simulink model "qbot2_post_processing"  (R2020a)
settings: Solver=FixedStepDiscrete  StartTime=0.0  StopTime=P.t(end)  FixedStep=P.dt  RelTol=1e-3  EnableMultiTasking=on
StopFcn:
  | plot_sim(out, P)
settings Model: ExtModeTrigDuration=10000  Creator=divad  LastModifiedBy=divad
settings SolverCC: PositivePriorityOrder=on
settings DataIOCC: SaveOutput=off  SignalLogging=off  DSMLogging=off  SaveTime=off
settings OptimizationCC: LifeSpan=inf
settings DebuggingCC: ArithmeticOperatorsInVariantConditions=warning
settings SFSimCC: SimUseLocalCustomCode=off  CustomCodeUndefinedFunction=UseInterfaceOnly
settings RTWCC: Description=QUARC Win64 Target  SystemTargetFile=quarc_win64.tlc  TemplateMakefile=quarc_default_tmf  RTWUseLocalCustomCode=off
settings CodeAppCC: StateflowObjectComments=on
settings STFCustomTargetCC: TargetPreCompLibLocation=C:\PROGRA~3\QUARC\lib\2020a\win64\release  TargetLangStandard=C99 (ISO)  ConcurrentExecutionCompliant=on  GRTInterface=on  SystemTargetFile=quarc_win64.tlc
settings GRTTargetCC: TargetPreCompLibLocation=C:\PROGRA~3\QUARC\lib\2020a\win64\release  ParMdlRefBuildCompliant=off  CompOptLevelCompliant=off  CombineOutputUpdateFcns=off  MatFileLogging=off  CPPClassGenCompliant=off  GRTInterface=on  UseToolchainInfoCompliant=off  ExtMode=on  ExtModeMexFile=quarc_comm
settings ConfigComp: CovMetricSettings=dswe

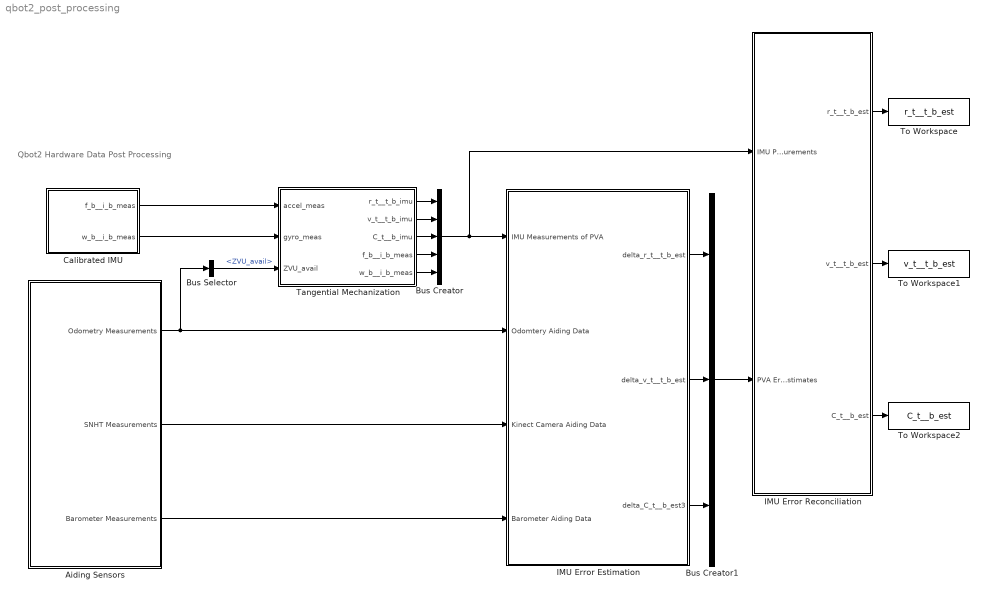
== system qbot2_post_processing ==
  note: Qbot2 Hardware Data Post Processing
  Aiding Sensors : Subsystem
  Bus Creator : BusCreator  Inputs=5
  Bus Creator1 : BusCreator  Inputs=3
  Bus Selector : BusSelector  OutputSignals=ZVU_avail
  Calibrated IMU : Subsystem
  IMU Error Estimation : Subsystem
  IMU Error Reconciliation : Subsystem
  Tangential Mechanization : Subsystem
  To Workspace : ToWorkspace  VariableName=r_t__t_b_est  SampleTime=-1
  To Workspace1 : ToWorkspace  VariableName=v_t__t_b_est  SampleTime=-1
  To Workspace2 : ToWorkspace  VariableName=C_t__b_est  SampleTime=-1
  wires:
  Calibrated IMU/1(f_b__i_b_meas) -> Tangential Mechanization/1(accel_meas)
  Calibrated IMU/2(w_b__i_b_meas) -> Tangential Mechanization/2(gyro_meas)
  Tangential Mechanization/1(r_t__t_b_imu) -> Bus Creator/1
  Tangential Mechanization/2(v_t__t_b_imu) -> Bus Creator/2
  Tangential Mechanization/3(C_t__b_imu) -> Bus Creator/3
  Tangential Mechanization/4(f_b__i_b_meas) -> Bus Creator/4
  Tangential Mechanization/5(w_b__i_b_meas) -> Bus Creator/5
  Bus Creator1/1 -> IMU Error Reconciliation/2(PVA Error Estimates)
  IMU Error Reconciliation/1(r_t__t_b_est) -> To Workspace/1
  IMU Error Reconciliation/2(v_t__t_b_est) -> To Workspace1/1
  IMU Error Reconciliation/3(C_t__b_est) -> To Workspace2/1
  Bus Creator/1 -> IMU Error Estimation/1(IMU Measurements of PVA), IMU Error Reconciliation/1(IMU PVA Measurements)
  Aiding Sensors/1(Odometry Measurements) -> Bus Selector/1, IMU Error Estimation/2(Odomtery Aiding Data)
  Aiding Sensors/2(SNHT Measurements) -> IMU Error Estimation/3(Kinect Camera Aiding Data)
  Aiding Sensors/3(Barometer Measurements) -> IMU Error Estimation/4(Barometer Aiding Data)
  IMU Error Estimation/2(delta_v_t__t_b_est) -> Bus Creator1/2
  IMU Error Estimation/3(delta_C_t__b_est3) -> Bus Creator1/3
  IMU Error Estimation/1(delta_r_t__t_b_est) -> Bus Creator1/1
  Bus Selector/1 -> Tangential Mechanization/3(ZVU_avail)  "<ZVU_avail>"

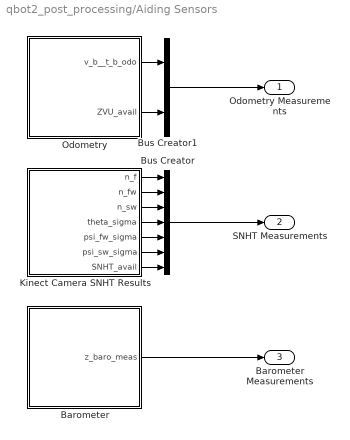
== system qbot2_post_processing/Aiding Sensors ==
  Barometer : Subsystem
  Bus Creator : BusCreator  Inputs=7
  Bus Creator1 : BusCreator  Inputs=2
  Kinect Camera SNHT Results : Subsystem
  Odometry : Subsystem
  Odometry Measurements : Outport
  SNHT Measurements : Outport  Port=2
  Barometer Measurements : Outport  Port=3
  wires:
  Odometry/2(ZVU_avail) -> Bus Creator1/2
  Bus Creator1/1 -> Odometry Measurements/1
  Odometry/1(v_b__t_b_odo) -> Bus Creator1/1
  Barometer/1(z_baro_meas) -> Barometer Measurements/1
  Kinect Camera SNHT Results/1(n_f) -> Bus Creator/1
  Kinect Camera SNHT Results/2(n_fw) -> Bus Creator/2
  Kinect Camera SNHT Results/3(n_sw) -> Bus Creator/3
  Kinect Camera SNHT Results/4(theta_sigma) -> Bus Creator/4
  Kinect Camera SNHT Results/5(psi_fw_sigma) -> Bus Creator/5
  Kinect Camera SNHT Results/6(psi_sw_sigma) -> Bus Creator/6
  Kinect Camera SNHT Results/7(SNHT_avail) -> Bus Creator/7
  Bus Creator/1 -> SNHT Measurements/1

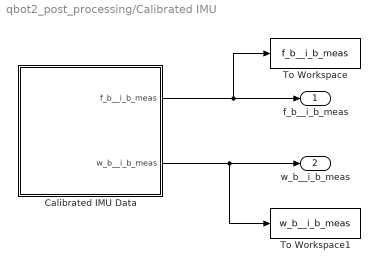
== system qbot2_post_processing/Calibrated IMU ==
  Calibrated IMU Data : MATLAB Function  TreatAsAtomicUnit=on
  To Workspace : ToWorkspace  VariableName=f_b__i_b_meas  SampleTime=-1
  To Workspace1 : ToWorkspace  VariableName=w_b__i_b_meas  SampleTime=-1
  f_b__i_b_meas : Outport
  w_b__i_b_meas : Outport  Port=2
  wires:
  Calibrated IMU Data/2(w_b__i_b_meas) -> To Workspace1/1, w_b__i_b_meas/1
  Calibrated IMU Data/1(f_b__i_b_meas) -> To Workspace/1, f_b__i_b_meas/1

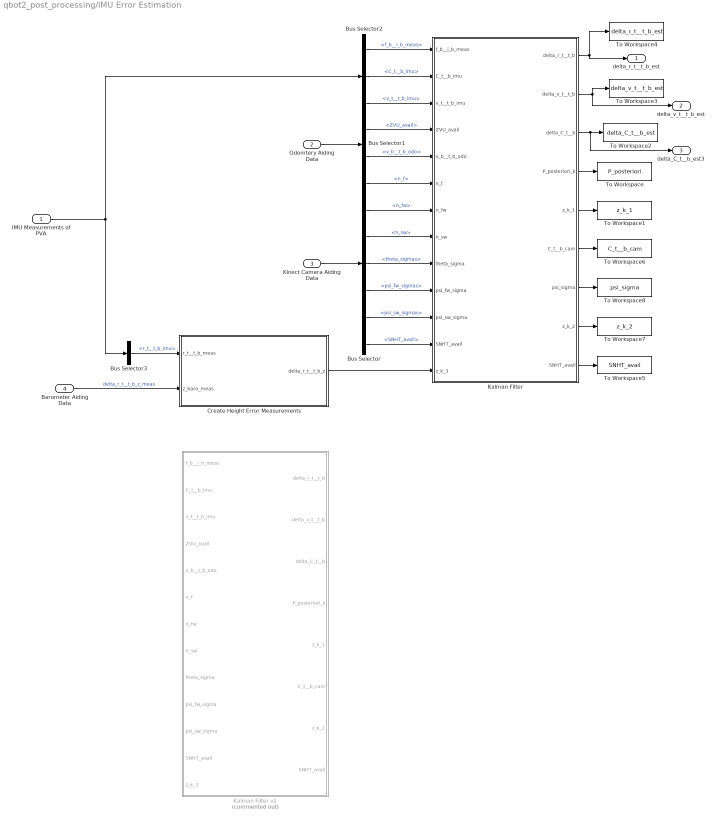
== system qbot2_post_processing/IMU Error Estimation ==
  IMU Measurements of PVA : Inport
  Odomtery Aiding Data : Inport  Port=2
  Kinect Camera Aiding Data : Inport  Port=3
  Barometer Aiding Data : Inport  Port=4
  Bus Selector : BusSelector  OutputSignals=n_f,n_fw,n_sw,theta_sigmas,psi_fw_sigmas,psi_sw_sigmas,SNHT_avail
  Bus Selector1 : BusSelector  OutputSignals=ZVU_avail,v_b__t_b_odo
  Bus Selector2 : BusSelector  OutputSignals=f_b__i_b_meas,C_t__b_imu,v_t__t_b_imu
  Bus Selector3 : BusSelector  OutputSignals=r_t__t_b_imu
  Create Height Error Measurements : Subsystem
  Kalman Filter : MATLAB Function  TreatAsAtomicUnit=on
  Kalman Filter v2 : MATLAB Function  Commented=on  TreatAsAtomicUnit=on
  To Workspace : ToWorkspace  VariableName=P_posteriori  SampleTime=-1
  To Workspace1 : ToWorkspace  VariableName=z_k_1  SampleTime=-1
  To Workspace2 : ToWorkspace  VariableName=delta_C_t__b_est  SampleTime=-1
  To Workspace3 : ToWorkspace  VariableName=delta_v_t__t_b_est  SampleTime=-1
      settings: Save2DSignal=2-D array (concatenate along first dimension)
  To Workspace4 : ToWorkspace  VariableName=delta_r_t__t_b_est  SampleTime=-1
      settings: Save2DSignal=2-D array (concatenate along first dimension)
  To Workspace5 : ToWorkspace  VariableName=SNHT_avail  SampleTime=-1
      settings: Save2DSignal=2-D array (concatenate along first dimension)
  To Workspace6 : ToWorkspace  VariableName=C_t__b_cam  SampleTime=-1
  To Workspace7 : ToWorkspace  VariableName=z_k_2  SampleTime=-1
      settings: Save2DSignal=2-D array (concatenate along first dimension)
  To Workspace8 : ToWorkspace  VariableName=psi_sigma  SampleTime=-1
      settings: Save2DSignal=2-D array (concatenate along first dimension)
  delta_r_t__t_b_est : Outport
  delta_v_t__t_b_est : Outport  Port=2
  delta_C_t__b_est3 : Outport  Port=3
  wires:
  IMU Measurements of PVA/1 -> Bus Selector3/1, Bus Selector2/1
  Barometer Aiding Data/1 -> Create Height Error Measurements/2(z_baro_meas)  "delta_r_t__t_b_z_meas"
  Odomtery Aiding Data/1 -> Bus Selector1/1
  Kinect Camera Aiding Data/1 -> Bus Selector/1
  Bus Selector3/1 -> Create Height Error Measurements/1(r_t__t_b_meas)  "<r_t__t_b_imu>"
  Bus Selector2/1 -> Kalman Filter/1(f_b__i_b_meas)  "<f_b__i_b_meas>"
  Bus Selector2/2 -> Kalman Filter/2(C_t__b_imu)  "<C_t__b_imu>"
  Bus Selector2/3 -> Kalman Filter/3(v_t__t_b_imu)  "<v_t__t_b_imu>"
  Bus Selector1/1 -> Kalman Filter/4(ZVU_avail)  "<ZVU_avail>"
  Bus Selector1/2 -> Kalman Filter/5(v_b__t_b_odo)  "<v_b__t_b_odo>"
  Bus Selector/1 -> Kalman Filter/6(n_f)  "<n_f>"
  Bus Selector/2 -> Kalman Filter/7(n_fw)  "<n_fw>"
  Bus Selector/3 -> Kalman Filter/8(n_sw)  "<n_sw>"
  Bus Selector/4 -> Kalman Filter/9(theta_sigma)  "<theta_sigmas>"
  Bus Selector/5 -> Kalman Filter/10(psi_fw_sigma)  "<psi_fw_sigmas>"
  Bus Selector/6 -> Kalman Filter/11(psi_sw_sigma)  "<psi_sw_sigmas>"
  Bus Selector/7 -> Kalman Filter/12("SNHT_avail ")  "<SNHT_avail>"
  Create Height Error Measurements/1(delta_r_t__t_b_z) -> Kalman Filter/13(z_k_3)
  Kalman Filter/9(SNHT_avail) -> To Workspace5/1
  Kalman Filter/8(z_k_2) -> To Workspace7/1
  Kalman Filter/6(C_t__b_cam) -> To Workspace6/1
  Kalman Filter/5(z_k_1) -> To Workspace1/1
  Kalman Filter/4(P_posteriori_k) -> To Workspace/1
  Kalman Filter/3(delta_C_t__b) -> delta_C_t__b_est3/1, To Workspace2/1
  Kalman Filter/2(delta_v_t__t_b) -> delta_v_t__t_b_est/1, To Workspace3/1
  Kalman Filter/1(delta_r_t__t_b) -> To Workspace4/1, delta_r_t__t_b_est/1
  Kalman Filter/7(psi_sigma) -> To Workspace8/1

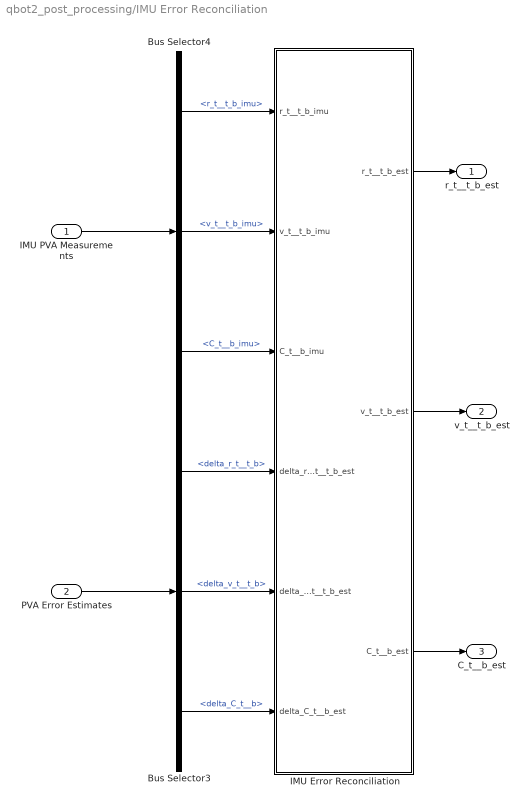
== system qbot2_post_processing/IMU Error Reconciliation ==
  IMU PVA Measurements : Inport
  PVA Error Estimates : Inport  Port=2
  Bus Selector3 : BusSelector  OutputSignals=delta_r_t__t_b,delta_v_t__t_b,delta_C_t__b
  Bus Selector4 : BusSelector  OutputSignals=r_t__t_b_imu,v_t__t_b_imu,C_t__b_imu
  IMU Error Reconciliation : MATLAB Function  TreatAsAtomicUnit=on
  r_t__t_b_est : Outport
  v_t__t_b_est : Outport  Port=2
  C_t__b_est : Outport  Port=3
  wires:
  Bus Selector3/1 -> IMU Error Reconciliation/4(delta_r_t__t_b_est)  "<delta_r_t__t_b>"
  IMU Error Reconciliation/3(C_t__b_est) -> C_t__b_est/1
  Bus Selector4/2 -> IMU Error Reconciliation/2(v_t__t_b_imu)  "<v_t__t_b_imu>"
  Bus Selector4/3 -> IMU Error Reconciliation/3(C_t__b_imu)  "<C_t__b_imu>"
  IMU PVA Measurements/1 -> Bus Selector4/1
  Bus Selector3/2 -> IMU Error Reconciliation/5(delta_v_t__t_b_est)  "<delta_v_t__t_b>"
  IMU Error Reconciliation/2(v_t__t_b_est) -> v_t__t_b_est/1
  Bus Selector4/1 -> IMU Error Reconciliation/1(r_t__t_b_imu)  "<r_t__t_b_imu>"
  Bus Selector3/3 -> IMU Error Reconciliation/6(delta_C_t__b_est)  "<delta_C_t__b>"
  PVA Error Estimates/1 -> Bus Selector3/1
  IMU Error Reconciliation/1(r_t__t_b_est) -> r_t__t_b_est/1

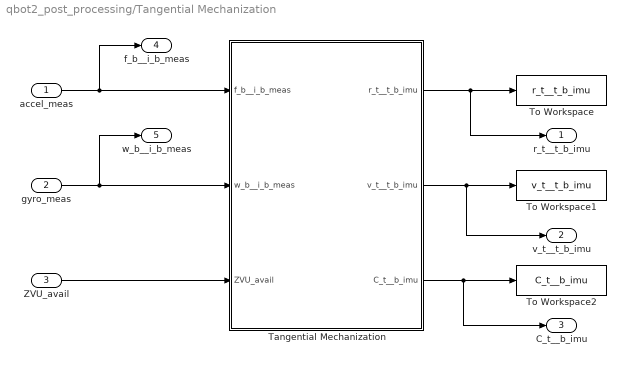
== system qbot2_post_processing/Tangential Mechanization ==
  accel_meas : Inport
  gyro_meas : Inport  Port=2
  ZVU_avail : Inport  Port=3
  Tangential Mechanization : MATLAB Function  TreatAsAtomicUnit=on
  To Workspace : ToWorkspace  VariableName=r_t__t_b_imu  SampleTime=-1
      settings: Save2DSignal=2-D array (concatenate along first dimension)
  To Workspace1 : ToWorkspace  VariableName=v_t__t_b_imu  SampleTime=-1
      settings: Save2DSignal=2-D array (concatenate along first dimension)
  To Workspace2 : ToWorkspace  VariableName=C_t__b_imu  SampleTime=-1
  r_t__t_b_imu : Outport
  v_t__t_b_imu : Outport  Port=2
  C_t__b_imu : Outport  Port=3
  f_b__i_b_meas : Outport  Port=4
  w_b__i_b_meas : Outport  Port=5
  wires:
  Tangential Mechanization/3(C_t__b_imu) -> C_t__b_imu/1, To Workspace2/1
  Tangential Mechanization/2(v_t__t_b_imu) -> v_t__t_b_imu/1, To Workspace1/1
  gyro_meas/1 -> Tangential Mechanization/2(w_b__i_b_meas), w_b__i_b_meas/1
  Tangential Mechanization/1(r_t__t_b_imu) -> r_t__t_b_imu/1, To Workspace/1
  accel_meas/1 -> Tangential Mechanization/1(f_b__i_b_meas), f_b__i_b_meas/1
  ZVU_avail/1 -> Tangential Mechanization/3(ZVU_avail)

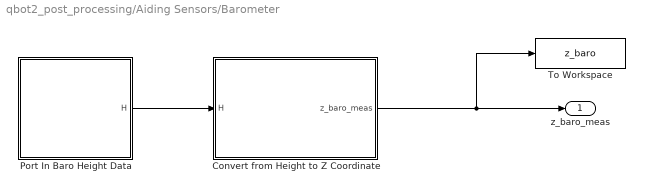
== system qbot2_post_processing/Aiding Sensors/Barometer ==
  Convert from Height to Z Coordinate : MATLAB Function  TreatAsAtomicUnit=on
  Port In Baro Height Data : MATLAB Function  TreatAsAtomicUnit=on
  To Workspace : ToWorkspace  VariableName=z_baro  SampleTime=-1
  z_baro_meas : Outport
  wires:
  Port In Baro Height Data/1(H) -> Convert from Height to Z Coordinate/1(H)
  Convert from Height to Z Coordinate/1(z_baro_meas) -> To Workspace/1, z_baro_meas/1

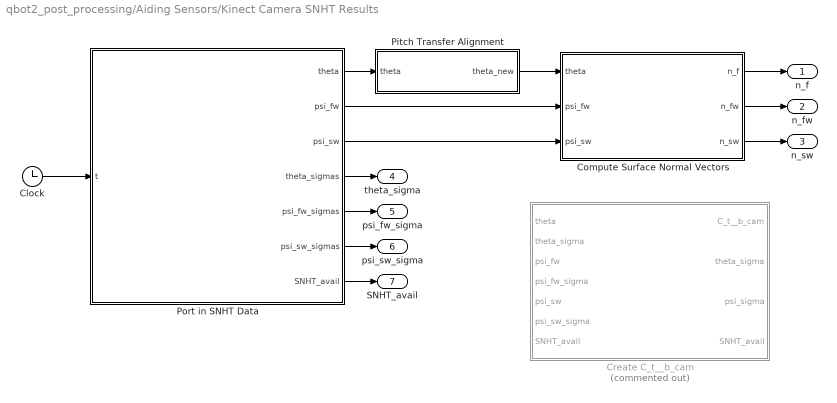
== system qbot2_post_processing/Aiding Sensors/Kinect Camera SNHT Results ==
  Clock : Clock
  Compute Surface Normal Vectors : MATLAB Function  TreatAsAtomicUnit=on
  Create C_t__b_cam : MATLAB Function  Commented=on  TreatAsAtomicUnit=on
  Pitch Transfer Alignment : MATLAB Function  TreatAsAtomicUnit=on
  Port in SNHT Data : MATLAB Function  TreatAsAtomicUnit=on
  n_f : Outport
  n_fw : Outport  Port=2
  n_sw : Outport  Port=3
  theta_sigma : Outport  Port=4
  psi_fw_sigma : Outport  Port=5
  psi_sw_sigma : Outport  Port=6
  SNHT_avail : Outport  Port=7
  wires:
  Port in SNHT Data/1(theta) -> Pitch Transfer Alignment/1(theta)
  Clock/1 -> Port in SNHT Data/1(t)
  Pitch Transfer Alignment/1(theta_new) -> Compute Surface Normal Vectors/1(theta)
  Port in SNHT Data/2(psi_fw) -> Compute Surface Normal Vectors/2(psi_fw)
  Port in SNHT Data/3(psi_sw) -> Compute Surface Normal Vectors/3(psi_sw)
  Port in SNHT Data/7(SNHT_avail) -> SNHT_avail/1
  Port in SNHT Data/6(psi_sw_sigmas) -> psi_sw_sigma/1
  Port in SNHT Data/4(theta_sigmas) -> theta_sigma/1
  Compute Surface Normal Vectors/1(n_f) -> n_f/1
  Compute Surface Normal Vectors/2(n_fw) -> n_fw/1
  Compute Surface Normal Vectors/3(n_sw) -> n_sw/1
  Port in SNHT Data/5(psi_fw_sigmas) -> psi_fw_sigma/1

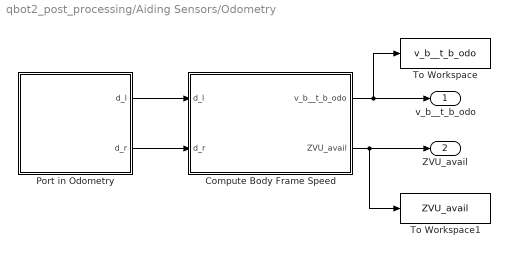
== system qbot2_post_processing/Aiding Sensors/Odometry ==
  Compute Body Frame Speed : MATLAB Function  TreatAsAtomicUnit=on
  Port in Odometry : MATLAB Function  TreatAsAtomicUnit=on
  To Workspace : ToWorkspace  VariableName=v_b__t_b_odo  SampleTime=-1
      settings: Save2DSignal=2-D array (concatenate along first dimension)
  To Workspace1 : ToWorkspace  VariableName=ZVU_avail  SampleTime=-1
  v_b__t_b_odo : Outport
  ZVU_avail : Outport  Port=2
  wires:
  Port in Odometry/2(d_r) -> Compute Body Frame Speed/2(d_r)
  Port in Odometry/1(d_l) -> Compute Body Frame Speed/1(d_l)
  Compute Body Frame Speed/2(ZVU_avail) -> To Workspace1/1, ZVU_avail/1
  Compute Body Frame Speed/1(v_b__t_b_odo) -> To Workspace/1, v_b__t_b_odo/1

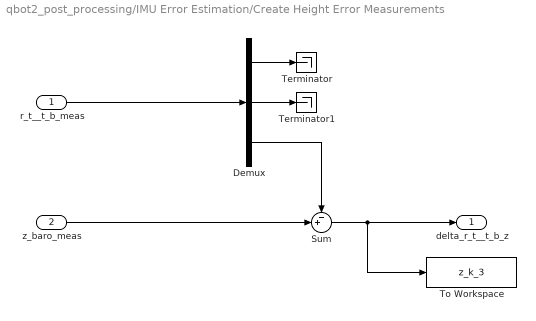
== system qbot2_post_processing/IMU Error Estimation/Create Height Error Measurements ==
  r_t__t_b_meas : Inport
  z_baro_meas : Inport  Port=2
  Demux : Demux  Outputs=3
  Sum : Sum  Inputs=-+|
  Terminator : Terminator
  Terminator1 : Terminator
  To Workspace : ToWorkspace  VariableName=z_k_3  SampleTime=-1
      settings: Save2DSignal=2-D array (concatenate along first dimension)
  delta_r_t__t_b_z : Outport
  wires:
  Demux/3 -> Sum/1
  Demux/2 -> Terminator1/1
  Demux/1 -> Terminator/1
  z_baro_meas/1 -> Sum/2
  Sum/1 -> To Workspace/1, delta_r_t__t_b_z/1
  r_t__t_b_meas/1 -> Demux/1

== matlab function qbot2_post_processing/IMU Error Estimation/Kalman Filter v2 ==
  data: f_b__i_b_meas input; C_t__b_imu input; v_t__t_b_imu input; ZVU_avail input; delta_r_t__t_b output; delta_v_t__t_b output; delta_C_t__b output; v_b__t_b_odo input; n_f input; n_fw input; n_sw input; theta_sigma input; psi_fw_sigma input; psi_sw_sigma input; SNHT_avail input; z_k_3 input; P parameter; P_posteriori_k output; z_k_1 output; C_t__b_cam output; z_k_2 output; SNHT_avail output
function [delta_r_t__t_b, delta_v_t__t_b, delta_C_t__b, P_posteriori_k, ...
          z_k_1, ...
          C_t__b_cam, z_k_2, SNHT_avail] = ...
          IMU_Error_State_Estimation(f_b__i_b_meas, C_t__b_imu, ...
                                     v_t__t_b_imu, ZVU_avail, v_b__t_b_odo, ...
                                     n_f, n_fw, n_sw, theta_sigma, psi_fw_sigma, psi_sw_sigma, SNHT_avail, ...
                                     z_k_3, ...
                                     P)

%% IMU Error State Estimation Function
% Recieves error measurements from the difference between odometry and the
% IMU, and provides estimates of that error.  

persistent x_posteriori_k_1 P_posteriori_k_1 A Q_bar

dt = P.dt;

%**************************************************************************
%% Kalman Filter Prediction Steps
%**************************************************************************

% For first instance only
if (isempty(x_posteriori_k_1))
    
    % Set Initial Values for x and P_______________________________________
    P_0 = diag([5 * pi/180; 5 * pi/180; 5 * pi/180; ... % Initial Attitude Uncertianty (Angle-Axis)
                0.5; 0.5; 0.5; ...                      % Initial Velocity Uncertianty
                0.25; 0.25; 0.25; ...                   % Initial Position Uncertianty 
                10 * P.sigma_n_accel; ...               % Initial Accel Bias Instability Uncertianty
                10 * P.sigma_n_gyro] .^ 2);             % Initial Gyro Bias Instability Uncertianty
            
    x_0 = [dcm2k(P.C_t__b_init); ...                    % First measurement of attitude 
           0; 0; 0;    ...                              % First measurement of velocity error
           0; 0; 0;    ...                              % {t} frame always starts at zero
           P.sigma_n_accel; ...                         % Initialize at the 1-sigma value
           P.sigma_n_gyro];                             % Initialize at the 1-sigma value
       
    x_posteriori_k_1 = x_0;
    P_posteriori_k_1 = P_0;
    
    % Build the Contiuous Time Model_______________________________________
    A = zeros(15, 15);
    
    % Compute A - Fifth Row
    A(13:15, 13:15) = -eye(3) ./ P.cor_time;
    
    % Compute A - Fourth Row
    A(10:12, 10:12) = -eye(3) ./ P.cor_time;
    
    % Compute A - Third Row
    A(7:9, 4:6) = eye(3);
    
    % Compute A - Second Row
    A(4:6, 1:3) = -vec2ss(C_t__b_imu * f_b__i_b_meas);
    A(4:6, 4:6) = -2 .* P.Ohm_t__i_e;
    A(4:6, 10:12) = -C_t__b_imu;

    % Compute the monstrosity A(4:6, 7:9) a.k.a. A_23
    r_e__e_b_hat = P.r_e__e_t; % initial position is always the origin
    [L_b_hat, ~, ~] = xyz2llh(r_e__e_b_hat, P);
    g_0 = Somigliana(L_b_hat, P);
    r_e__e_S = Geo_Radius(L_b_hat, P);
    A(4:6, 7:9) = P.C_e__t' * ((2 * g_0 * r_e__e_b_hat) / ...
                 (r_e__e_S * norm(r_e__e_b_hat)^2)) * ...
                  r_e__e_b_hat' * P.C_e__t;
    
    % Compute A - First Row
    A(1:3, 1:3) = -P.Ohm_t__i_e;
    A(1:3, 13:15) = -C_t__b_imu;
    
    % Define Q_bar_________________________________________________________
    Q_vec = [P.gyro_ARW.^2;   ...        % Attitude Process Noise rad/s
             P.accel_VRW.^2;  ...        % Velocity Process Noise m/s
             zeros(3,1);         ...     % Position Process Noise
             P.sigma_n_accel.^2; ...     % Accel Bias Instability Process Noise m/s
             P.sigma_n_gyro.^2];         % Gyro  Bias Instability Process Noise rad/s
     
    % Allow for a margin of error for tuning     
    Q_fudge_factor = 1;
    
    % Set Q
    Q_bar = diag(Q_fudge_factor .* Q_vec');
    
    % Discritize the Continuous Time Model_________________________________
    F = eye(15) + A*dt;
    Q = (1/2) * ((F*Q_bar*F') + Q_bar) * dt;
    
    % Compute first prediction_____________________________________________
    x_priori_k = F * x_0;
    P_priori_k = (F * P_0 * F') + Q;
    
%__________________________________________________________________________
% All other instances: State Prediction  
else
    
    % Re-compute the time varying arguements of A__________________________

    % Compute A - Second Row
    A(4:6, 1:3) = -vec2ss(C_t__b_imu * f_b__i_b_meas);
    A(4:6, 10:12) = -C_t__b_imu;
    
    % Compute A - First Row
    A(1:3, 13:15) = -C_t__b_imu;
    
    % Discritize the Continuous Time Model_________________________________
    F = eye(15) + A*dt;
    Q = (1/2) * ((F*Q_bar*F') + Q_bar) * dt;
    
    % Compute prediction step
    x_priori_k = (F * x_posteriori_k_1);
    P_priori_k = (F * P_posteriori_k_1 * F') + Q;
    
    % Symmetrisize P
    P_priori_k = (P_priori_k + P_priori_k') / 2;
    
end

%**************************************************************************
%% Compute Kalman Filter Measurements
%**************************************************************************

%__________________________________________________________________________
% Odometry Velocity Error Mesaurement Computation

if (P.aiding_sensor_config == 4) | ...
   (P.aiding_sensor_config == 6) | ...
   (P.aiding_sensor_config == 7)
    
    %- - - - - - - - - - - - - - - - - - - - - - - - - - - - - - - - - - -
    % If a Zero Velocity Update (ZVU) is available
    if (ZVU_avail == 1)
        
        % Then error is simply the measurement
        z_k_1 = -v_t__t_b_imu;
        
        % Uncertianty of Velocity Error is 5 millameters
        R_odo_vec = [0.001, 0.001, 0.001] .^ 2;     
    
    %- - - - - - - - - - - - - - - - - - - - - - - - - - - - - - - - - - - 
    % If a Zero Velocity is NOT Available
    else
        
        % Rotate v_b__t_b_odo with best estimate of attitude
        delta_C_t__b_est = k2dcm(x_priori_k(1:3,1));
        C_t__b_est = C_t__b_imu * delta_C_t__b_est';
        v_t__t_b_odo = C_t__b_est * v_b__t_b_odo;
        delta_v_t__t_b_meas = v_t__t_b_odo - v_t__t_b_imu;
        z_k_1 = delta_v_t__t_b_meas;
        
        % Define R Vector
        R_b_vec = [0.05, 0.01, 0.01] .^ 2;   % Will come back to this!
        
        % Build the R Matrix
        R_odo = C_t__b_imu * diag(R_b_vec) * C_t__b_imu';
        R_odo_vec = [R_odo(1,1), R_odo(2,2), R_odo(3,3)];
        
    end

else
    
    z_k_1 = zeros(3,1);
 
end

%__________________________________________________________________________
% Kinect Camera Attitude Error Measurement Computation

if ((P.aiding_sensor_config == 5) | ...
    (P.aiding_sensor_config == 6) | ...
    (P.aiding_sensor_config == 7))
    
    if (SNHT_avail == 1)
        
        % Compute C_t__b_est
        delta_C_t__b_est = k2dcm(x_priori_k(1:3,1));
        C_t__b_est = C_t__b_imu * delta_C_t__b_est';
        
        % Compute C_t__b_cam
        [C_t__b_cam, psi_sigma, SNHT_avail] = get_C_t__b_cam(n_f, n_fw, n_sw, ...
            psi_fw_sigma, psi_sw_sigma, C_t__b_imu, C_t__b_est);
        
        if (SNHT_avail == 1)
            
            % Define R_e with known sigmas
            R_e = diag([1 * pi/180, theta_sigma, psi_sigma]) .^ 2;
            
            % Create Error in Attitude Measurement
            z_k_2 = dcm2k(C_t__b_cam * C_t__b_imu');
            
            % Compute Jacobian
            [~, pitch, roll] = dcm2ypr(C_t__b_est);
            J = [1, 0, -sin(pitch); ...
                0, cos(roll), sin(roll)*cos(pitch); ...
                0, -sin(roll), cos(roll)*cos(pitch)];
            
            % Convert R_e to R_k
            R_k = J * R_e * J';
            R_k_vec = [R_k(1), R_k(2), R_k(3)];
            
        else
            
            z_k_2 = zeros(3,1);
            R_k_vec = zeros(1,3);
            C_t__b_cam = eye(3);
            
        end
        
        
    else
        
        z_k_2 = zeros(3,1);
        R_k_vec = zeros(1,3);
        C_t__b_cam = eye(3);
        
    end
    
else
    
    z_k_2 = zeros(3,1);
    R_k_vec = zeros(1,3);
    C_t__b_cam = eye(3);
    
end

%**************************************************************************
%% Kalman Filter Measurement Update Steps
%**************************************************************************
% This section is segmented according to the aiding sensor configuration

%__________________________________________________________________________
% If no aiding sensors are included
if (P.aiding_sensor_config == 0)
    
    x_posteriori_k = x_priori_k;
    P_posteriori_k = P_priori_k;

%__________________________________________________________________________
% If any aiding sensor is selected
else
    
    % Create Starting Point
    H = zeros(9,15);
    R_vec = 10^6 * ones(1,9);
    z = zeros(9,1);
    
    % Build H & R & z for Odometry
    if (P.aiding_sensor_config ~= 5)
        if (norm(x_priori_k) <= (10 * pi/180))
            H(4:6,:) = [vec2ss(v_t__t_b_imu), eye(3), zeros(3,9)];
        else
            H(4:6,:) = [zeros(3,3), eye(3), zeros(3,9)];
        end
        R_vec(4:6) = R_odo_vec;
        z(4:6) = z_k_1;
    end
    
    % Build H & R & z for Kinect Camera if present
    if (SNHT_avail == 1)
        H(1:3,:) = [eye(3), zeros(3,12)];
        R_vec(1:3) = R_k_vec;
        z(1:3) = z_k_2;
    end
    
    
    % Build H & R & z for Barometer is present
    if (P.aiding_sensor_config == 7)
        H(9,9) = 1;
        R_vec(9) = 0.3^2;
        z(9) = z_k_3;
    end
    
    
    % Build full R
    R = diag(R_vec);
    
    % Complete full measurement update
    % Kalman Gain Computation
    K = (P_priori_k * H') / (H * P_priori_k * H' + R);
    
    % A Posteriori State and Covariance Update
    x_posteriori_k = x_priori_k + K*(z - H*x_priori_k);
    P_posteriori_k = (eye(15) - K*H) * P_priori_k;
    
    %Symmetrisize P
    P_posteriori_k = (P_posteriori_k + P_posteriori_k') / 2;
    
end

%__________________________________________________________________________
%% Pick-off State Estimates for Function Output

% State Estimates (AVP -> PVA)
delta_x_t__t_b_est = [x_posteriori_k(7:9); ...
                      x_posteriori_k(4:6); ...
                      x_posteriori_k(1:3)];

% Pull Off Position, Velocity, and Attitude Error Separately
delta_r_t__t_b = delta_x_t__t_b_est(1:3);
delta_v_t__t_b = delta_x_t__t_b_est(4:6);
delta_k_t__t_b = delta_x_t__t_b_est(7:9);

% Create and Normalize delta_C_t__b
delta_C_t__b = k2dcm(delta_k_t__t_b);
delta_C_t__b = q2dcm(dcm2q(delta_C_t__b));

%__________________________________________________________________________
%% Save State Estimates for Next Loop

x_posteriori_k_1 = x_posteriori_k;
P_posteriori_k_1 = P_posteriori_k;

end

== matlab function qbot2_post_processing/Aiding Sensors/Kinect Camera SNHT Results/Port in SNHT Data ==
  data: t input; theta output; psi_fw output; psi_sw output; theta_sigmas output; psi_fw_sigmas output; psi_sw_sigmas output; P parameter; SNHT_avail output
function [theta, psi_fw, psi_sw, theta_sigmas, psi_fw_sigmas, psi_sw_sigmas, SNHT_avail] = port_in_SNHT(t, P)

%% Initialize
 persistent k
 
 if (isempty(k))
     k = 1;
 end
 
 %% Port in SNHT Results at 1 Hz
 
 if (mod(t, 1) == 0)
     
     % Pitch Results
     theta = P.theta_meas(k);
     theta_sigmas = P.theta_sigmas(k);
     
     % Front Wall Results
     psi_fw = P.psi_fw_meas(k);
     psi_fw_sigmas = P.psi_fw_sigmas(k);
     
     % Side Wall Results
     psi_sw = P.psi_sw_meas(k);
     psi_sw_sigmas = P.psi_sw_sigmas(k);
     
     % Make SNHT_avail true
     SNHT_avail = 1;
     
     % Increment
     k = k + 1;
     
 else
     
     % Pitch Results
     theta = P.pitch_trans_align;
     theta_sigmas = 45 * pi/180;
     
     % Front Wall Results
     psi_fw = 0;
     psi_fw_sigmas = 45 * pi/180;
     
     % Side Wall Results
     psi_sw = 90;
     psi_sw_sigmas = 45 * pi/180;
     
     % Make SNHT_avail true
     SNHT_avail = 0;
     
 end

 if (t == 0)
     SNHT_avail = 0;
 end

== matlab function qbot2_post_processing/Aiding Sensors/Kinect Camera SNHT Results/Create C_t__b_cam ==
  data: theta input; theta_sigma input; C_t__b_cam output; psi_fw input; psi_fw_sigma input; psi_sw input; psi_sw_sigma input; theta_sigma output; psi_sigma output; SNHT_avail input; SNHT_avail output
function [C_t__b_cam, theta_sigma, psi_sigma, SNHT_avail]  = ...
    create_C_t__b_cam(theta, theta_sigma, psi_fw, psi_fw_sigma, psi_sw, psi_sw_sigma, SNHT_avail)

%% Initialize Caresian Frame Axes
persistent x_b y_b z_b

if (isempty(x_b))
    
    % Define Body Frame Axes
    x_b = [1; 0; 0];
    y_b = [0; 1; 0];
    z_b = [0; 0; 1];
    
end

%% Only Complete when SNHT Results are available
if (SNHT_avail == 1)
    
    % Define normal vectors
    n_f  = [sin(theta); 0; cos(theta)];
    n_fw = [cos(psi_fw); sin(psi_fw); 0];
    n_sw = [-cos(psi_sw); sin(psi_sw); 0];
    
    % Normalize the Normal Vectors
    n_f = n_f / norm(n_f);
    n_fw = n_fw / norm(n_fw);
    n_sw = n_sw / norm(n_sw);
    
    % Define Body Frame Axes from Measurements, and Return Sigmas
    if (psi_fw_sigma <= psi_sw_sigma)
        x_t = n_fw;
        y_t = -(cross(n_fw, n_f));
        z_t = n_f;
        psi_sigma = psi_fw_sigma;
    else
        x_t = cross(n_sw, n_f);
        y_t = n_sw;
        z_t = n_f;
        psi_sigma = psi_sw_sigma;
    end
    
    %% Create C_t__b_cam
    
    % Build DCM
    C_b__t_cam = [dot(x_t, x_b), dot(y_t, x_b), dot(z_t, x_b); ...
                  dot(x_t, y_b), dot(y_t, y_b), dot(z_t, y_b); ...
                  dot(x_t, z_b), dot(y_t, z_b), dot(z_t, z_b)];
    
    C_t__b_cam = C_b__t_cam';
              
    % Normalize
    C_t__b_cam = q2dcm(dcm2q(C_t__b_cam));        

%% When SNHT Result is not Available
else
    
    % Set to default values
    C_t__b_cam = eye(3);
    theta_sigma = 45;
    psi_sigma = 45;
    
end

end

== matlab function qbot2_post_processing/Aiding Sensors/Barometer/Port In Baro Height Data ==
  data: H output; P parameter
function H = port_in_baro_data(P)

%% Initialize
persistent k T_s k_T p_s R g_0

if (isempty(k))
    
    % Initialize k
    k = 1;
    
    % Initialize Pressure to Height Conversion
    T_s = 288.15;
    k_T = 0.0065;
    p_s = 101.325;
    R = 287.058;
    g_0 = 9.0665;

end

%% Convert Pressure to Height
H = (T_s / k_T) * ((P.baro(k)/p_s)^(-R*k_T/g_0) - 1);

% Increment
k = k + 1;

end

== matlab function qbot2_post_processing/Aiding Sensors/Barometer/Convert from Height to Z Coordinate ==
  data: H input; z_baro_meas output; P parameter
function z_baro_meas = convert_H_to_z(H, P)

z_baro_meas = H - P.H_avg;

== matlab function qbot2_post_processing/Aiding Sensors/Kinect Camera SNHT Results/Pitch Transfer Alignment ==
  data: theta input; theta_new output; P parameter
function theta_new  = pitch_transfer_alignment(theta, P)

theta_new = theta - P.pitch_trans_align;

== matlab function qbot2_post_processing/IMU Error Reconciliation/IMU Error Reconciliation ==
  data: r_t__t_b_imu input; r_t__t_b_est output; v_t__t_b_imu input; C_t__b_imu input; v_t__t_b_est output; C_t__b_est output; delta_r_t__t_b_est input; delta_v_t__t_b_est input; delta_C_t__b_est input; P parameter
function [r_t__t_b_est, v_t__t_b_est, C_t__b_est] = ...
    imu_error_reconcile(r_t__t_b_imu, v_t__t_b_imu, C_t__b_imu, ...
                        delta_r_t__t_b_est, delta_v_t__t_b_est, delta_C_t__b_est, P)
       
% No reconciliation for pure imu only
if (P.aiding_sensor_config == 0)
    
    r_t__t_b_est = r_t__t_b_imu;
    v_t__t_b_est = v_t__t_b_imu;
    C_t__b_est = C_t__b_imu;

% Adjust for every other aiding sensor config
else
                    
    % Reconclie Position
    r_t__t_b_est = r_t__t_b_imu + delta_r_t__t_b_est;
    
    % Reconcile Velocity
    v_t__t_b_est = v_t__t_b_imu + delta_v_t__t_b_est;
    
    % Reconclie Attitude
    C_t__b_est = C_t__b_imu * delta_C_t__b_est;

end

== matlab function qbot2_post_processing/Aiding Sensors/Kinect Camera SNHT Results/Compute Surface Normal Vectors ==
  data: theta input; n_f output; psi_fw input; psi_sw input; n_fw output; n_sw output
function [n_f, n_fw, n_sw] = compute_surface_normal_vectors(theta, psi_fw, psi_sw)

% Build Normal Vectors
n_f = [sin(theta); 0; cos(theta)];
n_fw = [cos(psi_fw); sin(psi_fw); 0];
n_sw = [-cos(psi_sw); sin(psi_sw); 0];

end

== matlab function qbot2_post_processing/Calibrated IMU/Calibrated IMU Data ==
  data: f_b__i_b_meas output; w_b__i_b_meas output; P parameter
function [f_b__i_b_meas, w_b__i_b_meas] = IMU_meas(P)

persistent k

if (isempty(k))
    k = 1;
end

% Load Accel Frame
f_b__i_b_meas = P.f_b__i_b_meas(:,k);

% Load Gyro Frame
w_b__i_b_meas = P.w_b__i_b_meas(:,k);

% Index to Next Frame
k = k + 1;

== matlab function qbot2_post_processing/IMU Error Estimation/Kalman Filter ==
  data: f_b__i_b_meas input; C_t__b_imu input; v_t__t_b_imu input; ZVU_avail input; delta_r_t__t_b output; delta_v_t__t_b output; delta_C_t__b output; v_b__t_b_odo input; n_f input; n_fw input; n_sw input; theta_sigma input; psi_fw_sigma input; psi_sw_sigma input; SNHT_avail input; z_k_3 input; P parameter; P_posteriori_k output; z_k_1 output; C_t__b_cam output; psi_sigma output; z_k_2 output; SNHT_avail output
function [delta_r_t__t_b, delta_v_t__t_b, delta_C_t__b, P_posteriori_k, ...
          z_k_1, ...
          C_t__b_cam, psi_sigma, z_k_2, SNHT_avail] = ...
          IMU_Error_State_Estimation(f_b__i_b_meas, C_t__b_imu, ...
                                     v_t__t_b_imu, ZVU_avail, v_b__t_b_odo, ...
                                     n_f, n_fw, n_sw, theta_sigma, psi_fw_sigma, psi_sw_sigma, SNHT_avail, ...
                                     z_k_3, ...
                                     P)

%% IMU Error State Estimation Function
% Recieves error measurements from the difference between odometry and the
% IMU, and provides estimates of that error.  

persistent x_posteriori_k_1 P_posteriori_k_1 A Q_bar

dt = P.dt;

% Normalize C_t__b_est
C_t__b_imu = q2dcm(dcm2q(C_t__b_imu));

%**************************************************************************
%% Kalman Filter Prediction Steps
%**************************************************************************

% For first instance only
if (isempty(x_posteriori_k_1))
    
    % Set Initial Values for x and P_______________________________________
    P_0 = diag([5 * pi/180; 5 * pi/180; 5 * pi/180; ... % Initial Attitude Uncertianty (Angle-Axis)
                0.5; 0.5; 0.5; ...                      % Initial Velocity Uncertianty
                0.25; 0.25; 0.25; ...                   % Initial Position Uncertianty 
                10 * P.sigma_n_accel; ...               % Initial Accel Bias Instability Uncertianty
                10 * P.sigma_n_gyro] .^ 2);             % Initial Gyro Bias Instability Uncertianty
            
    x_0 = [dcm2k(P.C_t__b_init); ...                    % First measurement of attitude 
           0; 0; 0;    ...                              % First measurement of velocity error
           0; 0; 0;    ...                              % {t} frame always starts at zero
           P.sigma_n_accel; ...                         % Initialize at the 1-sigma value
           P.sigma_n_gyro];                             % Initialize at the 1-sigma value
       
    x_posteriori_k_1 = x_0;
    P_posteriori_k_1 = P_0;
    d_prev = 0;
    
    % Build the Contiuous Time Model_______________________________________
    A = zeros(15, 15);
    
    % Compute A - Fifth Row
    A(13:15, 13:15) = -eye(3) ./ P.cor_time;
    
    % Compute A - Fourth Row
    A(10:12, 10:12) = -eye(3) ./ P.cor_time;
    
    % Compute A - Third Row
    A(7:9, 4:6) = eye(3);
    
    % Compute A - Second Row
    A(4:6, 1:3) = -vec2ss(C_t__b_imu * f_b__i_b_meas);
    A(4:6, 4:6) = -2 .* P.Ohm_t__i_e;
    A(4:6, 10:12) = -C_t__b_imu;

    % Compute the monstrosity A(4:6, 7:9) a.k.a. A_23
    r_e__e_b_hat = P.r_e__e_t; % initial position is always the origin
    [L_b_hat, ~, ~] = xyz2llh(r_e__e_b_hat, P);
    g_0 = Somigliana(L_b_hat, P);
    r_e__e_S = Geo_Radius(L_b_hat, P);
    A(4:6, 7:9) = P.C_e__t' * ((2 * g_0 * r_e__e_b_hat) / ...
                 (r_e__e_S * norm(r_e__e_b_hat)^2)) * ...
                  r_e__e_b_hat' * P.C_e__t;
    
    % Compute A - First Row
    A(1:3, 1:3) = -P.Ohm_t__i_e;
    A(1:3, 13:15) = -C_t__b_imu;
    
    % Define Q_bar_________________________________________________________
    Q_vec = [P.gyro_ARW.^2;   ...        % Attitude Process Noise rad/s
             P.accel_VRW.^2;  ...        % Velocity Process Noise m/s
             zeros(3,1);         ...     % Position Process Noise
             P.sigma_n_accel.^2; ...     % Accel Bias Instability Process Noise m/s
             P.sigma_n_gyro.^2];         % Gyro  Bias Instability Process Noise rad/s
     
    % Allow for a margin of error for tuning     
    Q_fudge_factor = 1;
    
    % Set Q
    Q_bar = diag(Q_fudge_factor .* Q_vec');
    
    % Discritize the Continuous Time Model_________________________________
    F = eye(15) + A*dt;
    Q = (1/2) * ((F*Q_bar*F') + Q_bar) * dt;
    
    % Compute first prediction_____________________________________________
    x_priori_k = F * x_0;
    P_priori_k = (F * P_0 * F') + Q;
    
%__________________________________________________________________________
% All other instances: State Prediction  
else
    
    % Re-compute the time varying arguements of A__________________________

    % Compute A - Second Row
    A(4:6, 1:3) = -vec2ss(C_t__b_imu * f_b__i_b_meas);
    A(4:6, 10:12) = -C_t__b_imu;
    
    % Compute A - First Row
    A(1:3, 13:15) = -C_t__b_imu;
    
    % Discritize the Continuous Time Model_________________________________
    F = eye(15) + A*dt;
    Q = (1/2) * ((F*Q_bar*F') + Q_bar) * dt;
    
    % Compute prediction step
    x_priori_k = (F * x_posteriori_k_1);
    P_priori_k = (F * P_posteriori_k_1 * F') + Q;
    
    % Symmetrisize P
    P_priori_k = (P_priori_k + P_priori_k') / 2;
    
end

%**************************************************************************
%% Kalman Filter Measurement Update Steps
%**************************************************************************
% This section is segmented according to the aiding sensor configuration

%__________________________________________________________________________
% No Measurement Updates
if (P.aiding_sensor_config == 0)
    
    x_posteriori_k = x_priori_k;
    P_posteriori_k = P_priori_k;
    
end

%__________________________________________________________________________
% Odometry Aiding 
if (P.aiding_sensor_config == 4) | ...
   (P.aiding_sensor_config == 6) | ...
   (P.aiding_sensor_config == 7)

    %- - - - - - - - - - - - - - - - - - - - - - - - - - - - - - - - - - -
    % If a Zero Velocity Update (ZVU) is available
    if (ZVU_avail == 1)
        
        % Then error is simply the measurement
        z_k_1 = -v_t__t_b_imu;
        
        % Uncertianty of Velocity Error is 5 millameters
        R = diag([0.01, 0.01, 0.01]) .^ 2;              % might be too small?
        
        % Set H Matrix -- H = [(v_t__t_b,x), I_3, 0_3, 0_3, 0_3]
        if (norm(x_priori_k(1:3)) <= (0 * pi/180))
            H = [vec2ss(v_t__t_b_imu), eye(3), zeros(3,9)];
        else
            H = [zeros(3,3), eye(3), zeros(3,9)];
        end      

        % Kalman Gain Computation
        K = (P_priori_k * H') / (H * P_priori_k * H' + R);
        
        % A Posteriori State and Covariance Update
        x_posteriori_k = x_priori_k + K*(z_k_1 - H*x_priori_k);
        P_posteriori_k = (eye(15) - K*H) * P_priori_k;
        
        %Symmetrisize P
        P_posteriori_k = (P_posteriori_k + P_posteriori_k') / 2;
    
    %- - - - - - - - - - - - - - - - - - - - - - - - - - - - - - - - - - - 
    % If a Zero Velocity Update (ZVU) is NOT available
    else
        
        % Rotate v_b__t_b_odo with best estimate of attitude
        delta_C_t__b_est = k2dcm(x_priori_k(1:3,1));
        C_t__b_est = C_t__b_imu * delta_C_t__b_est';
        v_t__t_b_odo = C_t__b_est * v_b__t_b_odo;
        delta_v_t__t_b_meas = v_t__t_b_odo - v_t__t_b_imu;
        z_k_1 = delta_v_t__t_b_meas;
        
        % Set H Matrix -- H = [(v_t__t_b,x), I_3, 0_3, 0_3, 0_3]
        if (norm(dcm2k(C_t__b_est)) <= (0 * pi/180))
            H = [vec2ss(v_t__t_b_imu), eye(3), zeros(3,9)];
        else
            H = [zeros(3,3), eye(3), zeros(3,9)];
        end
        
        % Define R Vector
        R_b_vec = [0.09, 0.015, 0.015] .^ 2;   % Will come back to this!
        
        % Build the R Matrix
        R = C_t__b_imu * diag(R_b_vec) * C_t__b_imu';
        
        % Kalman Gain Computation
        K = (P_priori_k * H') / (H * P_priori_k * H' + R);
        
        % A Posteriori State and Covariance Update
        x_posteriori_k = x_priori_k + K*(z_k_1 - H*x_priori_k);
        P_posteriori_k = (eye(15) - K*H) * P_priori_k;
        
        %Symmetrisize P
        P_posteriori_k = (P_posteriori_k + P_posteriori_k') / 2;
        
    end
    
else
    z_k_1 = zeros(3,1);

end    

%__________________________________________________________________________
% Kinect Camera Attitude Aiding
if ((P.aiding_sensor_config == 5) | ...
    (P.aiding_sensor_config == 6) | ...
    (P.aiding_sensor_config == 7))
    
    % Only Update at a frequency of 1 Hz
    if (SNHT_avail == 1)
        
        if (P.aiding_sensor_config == 4) | ...
           (P.aiding_sensor_config == 6) | ...
           (P.aiding_sensor_config == 7)
            x_priori_k = x_posteriori_k;
            P_priori_k = P_posteriori_k;
        end
        
        % Compute C_t__b_est
        delta_C_t__b_est = k2dcm(x_priori_k(1:3,1));
        C_t__b_est = C_t__b_imu * delta_C_t__b_est';
        
        % Compute C_t__b_cam
        [C_t__b_cam, psi_sigma, SNHT_avail] = get_C_t__b_cam(n_f, n_fw, n_sw, ...
                                                             psi_fw_sigma, psi_sw_sigma, C_t__b_imu, C_t__b_est);
        
        % Define R_e with known sigmas
        R_e = diag([1 * pi/180, theta_sigma, psi_sigma]) .^ 2;
        
        % If measurement is not rejected as an outlier
        if (SNHT_avail == 1)
            
            % Create Error in Attitude Measurement
            z_k_2 = dcm2k(C_t__b_cam * C_t__b_imu');
            
            % Compute Jacobian
            [~, pitch, roll] = dcm2ypr(C_t__b_est);
            J = [1, 0, -sin(pitch); ...
                0, cos(roll), sin(roll)*cos(pitch); ...
                0, -sin(roll), cos(roll)*cos(pitch)];
            
            % Convert R_e to R_k
            R_k = J * R_e * J';
            
            % Set H Matrix -- H = [I_3, 0_3, 0_3, 0_3, 0_3]
            H = [eye(3), zeros(3,12)];
            
            % Kalman Gain Computation
            K = (P_priori_k * H') / (H * P_priori_k * H' + R_k);
            
            % A Posteriori State and Covariance Update
            x_posteriori_k = x_priori_k + K*(z_k_2 - H*x_priori_k);
            P_posteriori_k = (eye(15) - K*H) * P_priori_k;
            
            %Symmetrisize P
            P_posteriori_k = (P_posteriori_k + P_posteriori_k') / 2;
            
        else
            
            % Carry Through
            x_posteriori_k = x_priori_k;
            P_posteriori_k = P_priori_k;
            z_k_2 = zeros(3,1);
            C_t__b_cam = eye(3);
            psi_sigma = 45 * pi/180;
            
        end
    
    % No measurement update at this time step
    else
        
        % Carry Through
        x_posteriori_k = x_priori_k;
        P_posteriori_k = P_priori_k;
        z_k_2 = zeros(3,1);
        C_t__b_cam = eye(3);
        psi_sigma = 45 * pi/180;
       
    end    

else
    z_k_2 = zeros(3,1);
    C_t__b_cam = eye(3);
    psi_sigma = 45 * pi/180;
end

%__________________________________________________________________________
% Barometer Aiding
if (P.aiding_sensor_config == 7)
    
    % Set H
    H = zeros(1,15);
    H(9) = 1;
    
    % Build the R Matrix
    R = 0.3^2; % m
    
    % Kalman Gain Computation
    K = (P_priori_k * H') / (H * P_priori_k * H' + R);
    
    % A Posteriori State and Covariance Update
    x_posteriori_k = x_priori_k + K*(z_k_3 - H*x_priori_k);
    P_posteriori_k = (eye(15) - K*H) * P_priori_k;
    
    %Symmetrisize P
    P_posteriori_k = (P_posteriori_k + P_posteriori_k') / 2;
    
end

%__________________________________________________________________________
%% Pick-off State Estimates for Function Output

% State Estimates (AVP -> PVA)
delta_x_t__t_b_est = [x_posteriori_k(7:9); ...
                      x_posteriori_k(4:6); ...
                      x_posteriori_k(1:3)];

% Pull Off Position, Velocity, and Attitude Error Separately
delta_r_t__t_b = delta_x_t__t_b_est(1:3);
delta_v_t__t_b = delta_x_t__t_b_est(4:6);
delta_k_t__t_b = delta_x_t__t_b_est(7:9);

% Create and Normalize delta_C_t__b
delta_C_t__b = k2dcm(delta_k_t__t_b);
delta_C_t__b = q2dcm(dcm2q(delta_C_t__b));

%__________________________________________________________________________
%% Save State Estimates for Next Loop

x_posteriori_k_1 = x_posteriori_k;
P_posteriori_k_1 = P_posteriori_k;

end

== matlab function qbot2_post_processing/Tangential Mechanization/Tangential Mechanization ==
  data: f_b__i_b_meas input; r_t__t_b_imu output; w_b__i_b_meas input; ZVU_avail input; v_t__t_b_imu output; C_t__b_imu output; P parameter
function [r_t__t_b_imu, v_t__t_b_imu, C_t__b_imu] = tan_mech(f_b__i_b_meas, w_b__i_b_meas, ZVU_avail, P)

%% Provide Initial Conditions
persistent r_t__t_b_prev v_t__t_b_prev C_t__b_prev g_t__b

if (isempty(r_t__t_b_prev))
    
    % Provide Initial Conditions
    r_t__t_b_prev = zeros(3,1);  % always start at origin for {t} frame
    v_t__t_b_prev = zeros(3,1);  % known value from staying still for 10s
    C_t__b_prev = P.C_t__b_init; % computed from first measurements
    
    % Calculate and store the vector g_t__b
    r_e__e_b = P.r_e__e_t + P.C_e__t*r_t__t_b_prev;         % Compute r_e__e_b
    [L_b, lambda_b, h_b] = xyz2llh(r_e__e_b, P);            % Compute the lat, lon, and height
    g_n__b = [0; 0; gravity(L_b, h_b, P)];                  % Compute the acceleration due to gravity
    C_e__n = Lat_Lon_2C_e__n(L_b, lambda_b);                % Compute C_e__n
    g_e__b = C_e__n * g_n__b;                               % Compute the gravity of the body in the {e} frame
    g_t__b = P.C_e__t' * g_e__b;                            % Compute the gravity of the body in the {t} frame 
    
end

%% Compute C_t__b_meas

% if (ZVU_avail == 1)
%     w_b__i_b_meas = zeros(3,1);
% end

% Calculate w_t__t_b_imu
w_t__t_b_imu = C_t__b_prev*w_b__i_b_meas - P.C_e__t'*P.w_i__i_e;
        
% Catch for when w_t__t_b is super super small
if (norm(w_t__t_b_imu) < (5 * eps))
    C_t__b_imu = C_t__b_prev;
else
    C_t__b_imu = Rodrigues_k(w_t__t_b_imu * P.dt) * C_t__b_prev;
end

% Normalize C_t__b_meas
C_t__b_imu = q2dcm(dcm2q(C_t__b_imu));

%% Compute v_t__t_b_imu

if (ZVU_avail == 1)
    
    a_t__t_b = zeros(3,1);
    v_t__t_b_imu = zeros(3,1);

else
    
    % f_t__i_b Specific Force Update
    f_t__i_b = C_t__b_imu * f_b__i_b_meas;
    
    % a_t__t_b Acceleration Vector Update
    a_t__t_b = f_t__i_b + g_t__b - 2*P.Ohm_t__i_e*v_t__t_b_prev;
    
    % v_t__t_b Velocity Vector Update
    v_t__t_b_imu = v_t__t_b_prev + a_t__t_b*P.dt;
    
end

%% Compute r_t__t_b_meas

% r_t__t_b Position Vector Update
r_t__t_b_imu = r_t__t_b_prev + v_t__t_b_prev*P.dt + a_t__t_b*((P.dt^2)/2);

%% Save Current Values as Previous Values

r_t__t_b_prev = r_t__t_b_imu;
v_t__t_b_prev = v_t__t_b_imu;
C_t__b_prev = C_t__b_imu;

== matlab function qbot2_post_processing/Aiding Sensors/Odometry/Port in Odometry ==
  data: d_l output; d_r output; P parameter
function [d_l, d_r] = port_in_odo(P)

%% Initialize

persistent k 

if (isempty(k))
    k = 1;
end

%% Port in Odometry Data

d_l = P.odo(k,2);
d_r = P.odo(k,1);

k = k + 1;

== matlab function qbot2_post_processing/Aiding Sensors/Odometry/Compute Body Frame Speed ==
  data: v_b__t_b_odo output; ZVU_avail output; d_l input; d_r input; P parameter
function [v_b__t_b_odo, ZVU_avail] = provide_body_speed_meas(d_l, d_r, P)

%% Initialize
persistent d_l_prev d_r_prev v_l_prev v_r_prev

n_samples = 5;
zvu_vect = zeros(1, n_samples);
if (isempty(d_l_prev))
    d_l_prev = 0;
    d_r_prev = 0;
    v_l_prev = zeros(1,n_samples);
    v_r_prev = zeros(1,n_samples);
end

%% Compute Wheel Velocities
v_l = (d_l - d_l_prev) / P.dt;
v_r = (d_r - d_r_prev) / P.dt;

% Scoot Data
v_l_prev(2:n_samples) = v_l_prev(1:n_samples-1);
v_r_prev(2:n_samples) = v_r_prev(1:n_samples-1);
v_l_prev(1) = v_l;
v_r_prev(1) = v_r;

%% Determine Zero Velocity Update (ZVU) Availability

if (sum(v_l_prev == zvu_vect) == n_samples) & (sum(v_r_prev == zvu_vect) == n_samples)
    ZVU_avail = 1;
else
    ZVU_avail = 0;
end

% Don't send an ZVU in the following configurations
if (P.aiding_sensor_config == 0) | (P.aiding_sensor_config == 5)
    ZVU_avail = 0;
end

%% Compute Body Frame Speed
v_b__t_b_odo = [(v_l + v_r)/2; 0; 0];

%% Save Current Wheel Positions as Previous Wheel Positions
d_l_prev = d_l;
d_r_prev = d_r;
